simulink model "remus_comparison"  (R2023b)
settings: Solver=VariableStepAuto  StartTime=0.0  StopTime=40  RelTol=1e-3
libraries: simulink_extras x8, mssSimulink x1
settings Model: Creator=arnaud  LastModifiedBy=arnaud

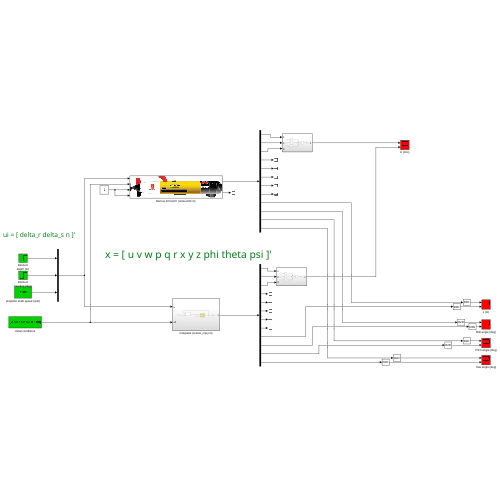
[thumbnail: Simulink's stored preview of the top-level diagram]
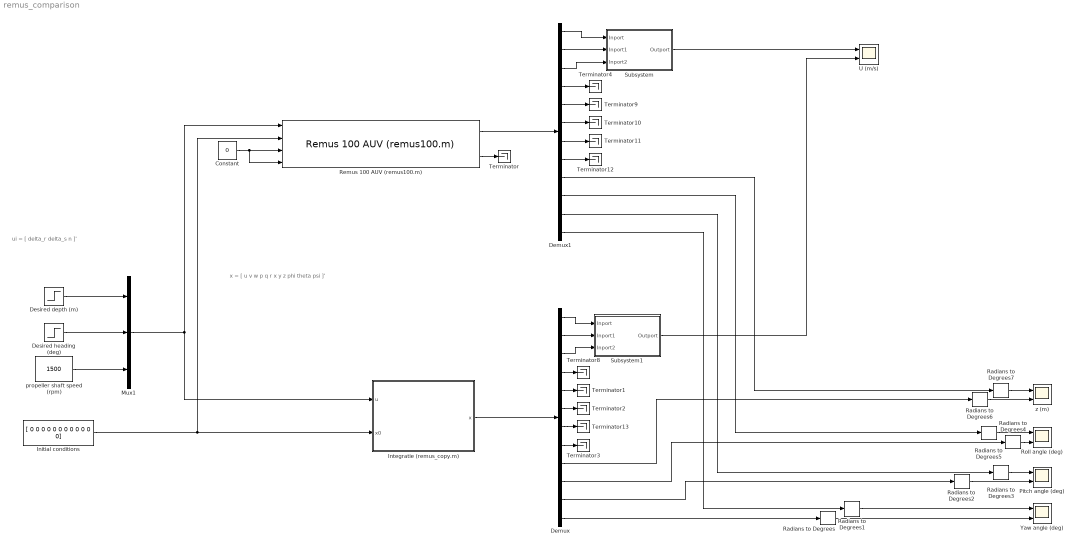
== system remus_comparison ==
  note: ui = [ delta_r delta_s n ]'
  note: x = [ u v w p q r x y z phi theta psi ]'
  Constant : Constant  Value=0
  Demux : Demux  Outputs=12
  Demux1 : Demux  Outputs=12
  Desired depth (m) : Step  Time=20  After=1.5*pi/180  SampleTime=0.05
  Desired heading (deg) : Step  Time=10  After=1.5*pi/180  SampleTime=0
  Initial conditions : Constant  Value="[ 0 0 0 0 0 0 0 0  0 0 0 0]"
  Integratie (remus_copy.m) : Subsystem
  Mux1 : Mux  Inputs=3
  Pitch angle (deg) : Scope  NumInputPorts=2
  Radians to Degrees{,1..7} (8 alike) : simulink_extras/Transformations/Radians to Degrees
  "Remus 100 AUV (remus100.m) " : mssSimulink/Marine craft models/Remus 100 AUV (remus100.m)  SystemSampleTime=-1  VariantActivationTime=update diagram  AllowFlexibleInterface=on  Latency=0  AutoFrameSizeCalculation=off
  Roll angle (deg) : Scope  NumInputPorts=2
  Subsystem : Subsystem
  Subsystem1 : Subsystem
  Terminator{,1..4,8..13} (11 alike) : Terminator
  U (m/s) : Scope  NumInputPorts=2
  Yaw angle (deg) : Scope  NumInputPorts=2
  propeller shaft speed (rpm) : Constant  Value=1500
  z (m) : Scope  NumInputPorts=2
  wires:
  Mux1/1 -> "Remus 100 AUV (remus100.m) "/1, Integratie (remus_copy.m)/1(u)
  Initial conditions/1 -> Integratie (remus_copy.m)/2(x0), "Remus 100 AUV (remus100.m) "/2
  Integratie (remus_copy.m)/1(x) -> Demux/1
  Constant/1 -> "Remus 100 AUV (remus100.m) "/3, "Remus 100 AUV (remus100.m) "/4
  "Remus 100 AUV (remus100.m) "/2 -> Terminator/1
  "Remus 100 AUV (remus100.m) "/1 -> Demux1/1
  Demux1/4 -> Terminator4/1
  Demux/12 -> Radians to Degrees/1
  Demux1/12 -> Radians to Degrees1/1
  Radians to Degrees/1 -> Yaw angle (deg)/2
  Radians to Degrees1/1 -> Yaw angle (deg)/1
  Radians to Degrees2/1 -> Pitch angle (deg)/2
  Radians to Degrees3/1 -> Pitch angle (deg)/1
  Demux/11 -> Radians to Degrees2/1
  Demux1/11 -> Radians to Degrees3/1
  Radians to Degrees4/1 -> Roll angle (deg)/2
  Radians to Degrees5/1 -> Roll angle (deg)/1
  Demux/10 -> Radians to Degrees4/1
  Demux1/10 -> Radians to Degrees5/1
  Demux/9 -> Radians to Degrees6/1
  Radians to Degrees6/1 -> z (m)/2
  Radians to Degrees7/1 -> z (m)/1
  Demux1/9 -> Radians to Degrees7/1
  Demux/2 -> Subsystem1/2(Inport1)
  Demux/1 -> Subsystem1/1(Inport)
  Demux/3 -> Subsystem1/3(Inport2)
  Demux/4 -> Terminator8/1
  Demux1/1 -> Subsystem/1(Inport)
  Demux1/2 -> Subsystem/2(Inport1)
  Demux1/3 -> Subsystem/3(Inport2)
  Subsystem/1(Outport) -> U (m/s)/1
  Demux1/8 -> Terminator12/1
  Demux1/7 -> Terminator11/1
  Demux1/5 -> Terminator9/1
  Demux1/6 -> Terminator10/1
  Demux/7 -> Terminator13/1
  Demux/8 -> Terminator3/1
  Demux/6 -> Terminator2/1
  Demux/5 -> Terminator1/1
  Subsystem1/1(Outport) -> U (m/s)/2
  propeller shaft speed (rpm)/1 -> Mux1/3
  Desired heading (deg)/1 -> Mux1/2
  Desired depth (m)/1 -> Mux1/1

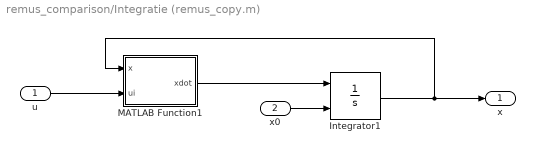
== system remus_comparison/Integratie (remus_copy.m) ==
  u : Inport
  x0 : Inport  Port=2
  Integrator1 : Integrator  InitialConditionSource=external  InitialCondition=[1 1]  UpperSaturationLimit=10  LowerSaturationLimit=-10
  MATLAB Function1 : MATLAB Function  TreatAsAtomicUnit=on
  x : Outport
  wires:
  u/1 -> MATLAB Function1/2(ui)
  Integrator1/1 -> x/1, MATLAB Function1/1(x)
  MATLAB Function1/1(xdot) -> Integrator1/1
  x0/1 -> Integrator1/2

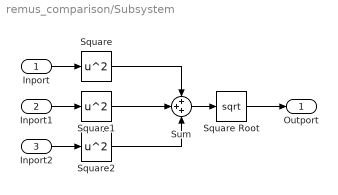
== system remus_comparison/Subsystem ==
  Inport : Inport
  Inport1 : Inport  Port=2
  Inport2 : Inport  Port=3
  Square : Math  Operator=square
  Square Root : Sqrt
  Square1 : Math  Operator=square
  Square2 : Math  Operator=square
  Sum : Sum  Inputs=+++
  Outport : Outport
  wires:
  Square/1 -> Sum/1
  Square Root/1 -> Outport/1
  Square1/1 -> Sum/2
  Inport/1 -> Square/1
  Inport2/1 -> Square2/1
  Inport1/1 -> Square1/1
  Sum/1 -> Square Root/1
  Square2/1 -> Sum/3

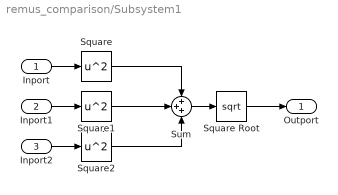
== system remus_comparison/Subsystem1 ==
  Inport : Inport
  Inport1 : Inport  Port=2
  Inport2 : Inport  Port=3
  Square : Math  Operator=square
  Square Root : Sqrt
  Square1 : Math  Operator=square
  Square2 : Math  Operator=square
  Sum : Sum  Inputs=+++
  Outport : Outport
  wires:
  Square/1 -> Sum/1
  Square Root/1 -> Outport/1
  Square1/1 -> Sum/2
  Inport/1 -> Square/1
  Inport2/1 -> Square2/1
  Inport1/1 -> Square1/1
  Sum/1 -> Square Root/1
  Square2/1 -> Sum/3

== matlab function remus_comparison/Integratie (remus_copy.m)/MATLAB Function1 ==
  data: x input; xdot output; ui input
function xdot = fcn(x,ui)

xdot = remus100_copy(x,ui);

end
